simulink library "RCD2"  (R2025b)
settings: Solver=VariableStepAuto  StartTime=0.0  StopTime=10.0  RelTol=1e-3
libraries: simulink x73, etargetslib x4, $bdroot x2
(part 2 of 2)

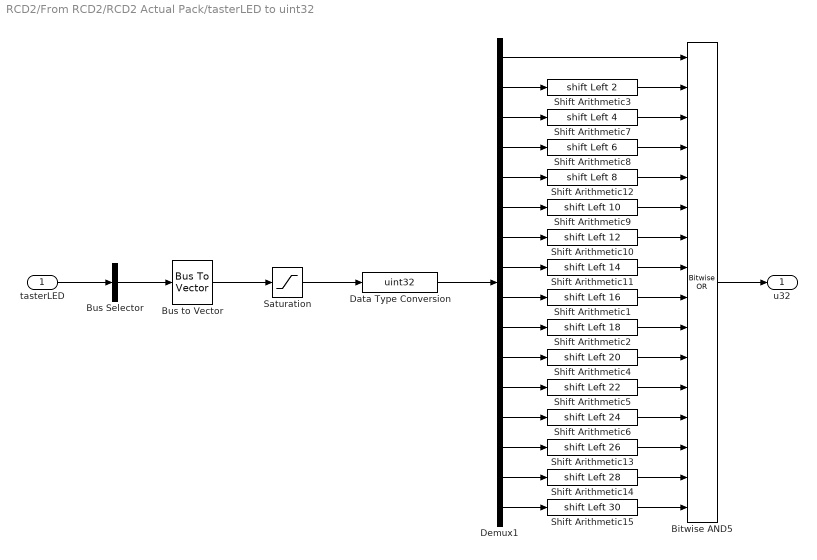
== system RCD2/From RCD2/RCD2 Actual Pack/tasterLED to uint32 ==
  "tasterLED " : Inport
  Bitwise AND5 : simulink/Logic and Bit Operations/Bitwise Operator  logicop=OR  UseBitMask=off  NumInputPorts=16  BitMask=bin2dec('11011001')  BitMaskRealWorld=Stored Integer
      settings: LibrarySourceBlock=|
      | simulink/Quick Insert/Logic and Bit
      | Operations/Bitwise AND
  Bus Selector : BusSelector  OutputSignals=tasterLED1,tasterLED2,tasterLED3,tasterLED4,tasterLED5,tasterLED6,tasterLED7,tasterLED8,tasterLED9,tasterLED10,tasterLED11,tasterLED12,tasterLED13,tasterLED14,tasterLED15,tasterLED16  OutputAsBus=on
  Bus to Vector : BusToVector
  Data Type Conversion : DataTypeConversion  OutDataTypeStr=uint32  SaturateOnIntegerOverflow=off  RndMeth=Floor
  Demux1 : Demux  Outputs=16
  Saturation : Saturate  UpperLimit=uint8(3)  LowerLimit=uint8(0)
  Shift Arithmetic1 : ArithShift  BitShiftNumber=16  BitShiftDirection=Left
  Shift Arithmetic10 : ArithShift  BitShiftNumber=12  BitShiftDirection=Left
  Shift Arithmetic11 : ArithShift  BitShiftNumber=14  BitShiftDirection=Left
  Shift Arithmetic12 : ArithShift  BitShiftNumber=8  BitShiftDirection=Left
  Shift Arithmetic13 : ArithShift  BitShiftNumber=26  BitShiftDirection=Left
  Shift Arithmetic14 : ArithShift  BitShiftNumber=28  BitShiftDirection=Left
  Shift Arithmetic15 : ArithShift  BitShiftNumber=30  BitShiftDirection=Left
  Shift Arithmetic2 : ArithShift  BitShiftNumber=18  BitShiftDirection=Left
  Shift Arithmetic3 : ArithShift  BitShiftNumber=2  BitShiftDirection=Left
  Shift Arithmetic4 : ArithShift  BitShiftNumber=20  BitShiftDirection=Left
  Shift Arithmetic5 : ArithShift  BitShiftNumber=22  BitShiftDirection=Left
  Shift Arithmetic6 : ArithShift  BitShiftNumber=24  BitShiftDirection=Left
  Shift Arithmetic7 : ArithShift  BitShiftNumber=4  BitShiftDirection=Left
  Shift Arithmetic8 : ArithShift  BitShiftNumber=6  BitShiftDirection=Left
  Shift Arithmetic9 : ArithShift  BitShiftNumber=10  BitShiftDirection=Left
  u32 : Outport
  wires:
  Bitwise AND5/1 -> u32/1
  Demux1/6 -> Shift Arithmetic9/1
  Demux1/5 -> Shift Arithmetic12/1
  Shift Arithmetic11/1 -> Bitwise AND5/8
  Shift Arithmetic10/1 -> Bitwise AND5/7
  Demux1/1 -> Bitwise AND5/1
  Shift Arithmetic9/1 -> Bitwise AND5/6
  Shift Arithmetic3/1 -> Bitwise AND5/2
  Demux1/8 -> Shift Arithmetic11/1
  Shift Arithmetic12/1 -> Bitwise AND5/5
  Shift Arithmetic7/1 -> Bitwise AND5/3
  Demux1/7 -> Shift Arithmetic10/1
  Demux1/3 -> Shift Arithmetic7/1
  Demux1/2 -> Shift Arithmetic3/1
  Demux1/4 -> Shift Arithmetic8/1
  Shift Arithmetic8/1 -> Bitwise AND5/4
  Demux1/9 -> Shift Arithmetic1/1
  Shift Arithmetic1/1 -> Bitwise AND5/9
  Demux1/10 -> Shift Arithmetic2/1
  Demux1/11 -> Shift Arithmetic4/1
  Shift Arithmetic2/1 -> Bitwise AND5/10
  Shift Arithmetic4/1 -> Bitwise AND5/11
  Demux1/12 -> Shift Arithmetic5/1
  Shift Arithmetic5/1 -> Bitwise AND5/12
  Demux1/13 -> Shift Arithmetic6/1
  Shift Arithmetic6/1 -> Bitwise AND5/13
  Shift Arithmetic13/1 -> Bitwise AND5/14
  Demux1/14 -> Shift Arithmetic13/1
  Shift Arithmetic14/1 -> Bitwise AND5/15
  Demux1/15 -> Shift Arithmetic14/1
  Shift Arithmetic15/1 -> Bitwise AND5/16
  Demux1/16 -> Shift Arithmetic15/1
  "tasterLED "/1 -> Bus Selector/1
  Bus Selector/1 -> Bus to Vector/1
  Bus to Vector/1 -> Saturation/1
  Data Type Conversion/1 -> Demux1/1
  Saturation/1 -> Data Type Conversion/1

== system RCD2/From RCD2/RCD2 Actual Unpack/Unpack Message ==
  bytes : Inport
  Enable : EnablePort
  Byte Unpack : etargetslib/Byte Unpack  dimensions={4,1,1,1,1,1,1,1,1,1,1,1}  datatypes={'uint8','uint8','double','single','single','single','single','single','single','uint16','uint32','uint16'}  byteAlign=1
      settings: LibrarySourceBlock=embeddedtargetslib/Host Communication/Byte Unpack
  CheckForValidProtocol : Subsystem
  Data Type Conversion{,1..5} (6 alike) : DataTypeConversion  OutDataTypeStr=double  SaturateOnIntegerOverflow=off  RndMeth=Floor
  Selector : Selector  IndexOptions=Index vector (dialog)  Indices=1:45  OutputSizes=1
  Subsystem : Subsystem
  u16 to bitfield : Subsystem
  u16 to tasterBitfield : Subsystem
  u32 to bitfield : Subsystem
  success : Outport
  busRCDActual : Outport  Port=2
  wires:
  bytes/1 -> Selector/1
  CheckForValidProtocol/1(isValid) -> success/1, Subsystem/Enable
  Subsystem/1(Out1) -> busRCDActual/1
  Data Type Conversion/1 -> Subsystem/2(In3)
  Data Type Conversion1/1 -> Subsystem/3(In4)
  Data Type Conversion2/1 -> Subsystem/4(In5)
  Data Type Conversion3/1 -> Subsystem/5(In6)
  Data Type Conversion4/1 -> Subsystem/6(In7)
  Data Type Conversion5/1 -> Subsystem/7(In8)
  u16 to tasterBitfield/1("tasterBitfield ") -> Subsystem/8(In9)
  u32 to bitfield/1("bitfield ") -> Subsystem/9(In10)
  u16 to bitfield/1("bitfield ") -> Subsystem/10(In11)
  Selector/1 -> Byte Unpack/1
  Byte Unpack/2 -> CheckForValidProtocol/2(headerID)
  Byte Unpack/1 -> CheckForValidProtocol/1(headerRCD)
  Byte Unpack/3 -> Subsystem/1(In1)
  Byte Unpack/4 -> Data Type Conversion/1
  Byte Unpack/5 -> Data Type Conversion1/1
  Byte Unpack/6 -> Data Type Conversion2/1
  Byte Unpack/7 -> Data Type Conversion3/1
  Byte Unpack/8 -> Data Type Conversion4/1
  Byte Unpack/9 -> Data Type Conversion5/1
  Byte Unpack/10 -> u16 to tasterBitfield/1(u16)
  Byte Unpack/11 -> u32 to bitfield/1(u32)
  Byte Unpack/12 -> u16 to bitfield/1(u16)

== system RCD2/To RCD2/RCD2 Command Pack/LED to uint16 ==
  "LED " : Inport
  Bitwise AND5 : simulink/Logic and Bit Operations/Bitwise Operator  logicop=OR  UseBitMask=off  NumInputPorts=8  BitMask=bin2dec('11011001')  BitMaskRealWorld=Stored Integer
      settings: LibrarySourceBlock=|
      | simulink/Quick Insert/Logic and Bit
      | Operations/Bitwise AND
  Bus Selector : BusSelector  OutputSignals=LED1,LED2,LED3,LED4,LED5,LED6,LED7,LED8  OutputAsBus=on
  Bus to Vector : BusToVector
  Data Type Conversion : DataTypeConversion  OutDataTypeStr=uint16  SaturateOnIntegerOverflow=off  RndMeth=Floor
  Demux1 : Demux  Outputs=8
  Saturation : Saturate  UpperLimit=uint8(3)  LowerLimit=uint8(0)
  Shift Arithmetic10 : ArithShift  BitShiftNumber=12  BitShiftDirection=Left
  Shift Arithmetic11 : ArithShift  BitShiftNumber=14  BitShiftDirection=Left
  Shift Arithmetic12 : ArithShift  BitShiftNumber=8  BitShiftDirection=Left
  Shift Arithmetic3 : ArithShift  BitShiftNumber=2  BitShiftDirection=Left
  Shift Arithmetic7 : ArithShift  BitShiftNumber=4  BitShiftDirection=Left
  Shift Arithmetic8 : ArithShift  BitShiftNumber=6  BitShiftDirection=Left
  Shift Arithmetic9 : ArithShift  BitShiftNumber=10  BitShiftDirection=Left
  u16 : Outport
  wires:
  Shift Arithmetic8/1 -> Bitwise AND5/4
  Demux1/4 -> Shift Arithmetic8/1
  Demux1/2 -> Shift Arithmetic3/1
  Demux1/3 -> Shift Arithmetic7/1
  Demux1/7 -> Shift Arithmetic10/1
  Shift Arithmetic7/1 -> Bitwise AND5/3
  Shift Arithmetic12/1 -> Bitwise AND5/5
  Demux1/8 -> Shift Arithmetic11/1
  Shift Arithmetic3/1 -> Bitwise AND5/2
  Shift Arithmetic9/1 -> Bitwise AND5/6
  Demux1/1 -> Bitwise AND5/1
  Shift Arithmetic10/1 -> Bitwise AND5/7
  Shift Arithmetic11/1 -> Bitwise AND5/8
  Demux1/5 -> Shift Arithmetic12/1
  Demux1/6 -> Shift Arithmetic9/1
  Bitwise AND5/1 -> u16/1
  "LED "/1 -> Bus Selector/1
  Bus Selector/1 -> Bus to Vector/1
  Bus to Vector/1 -> Saturation/1
  Data Type Conversion/1 -> Demux1/1
  Saturation/1 -> Data Type Conversion/1

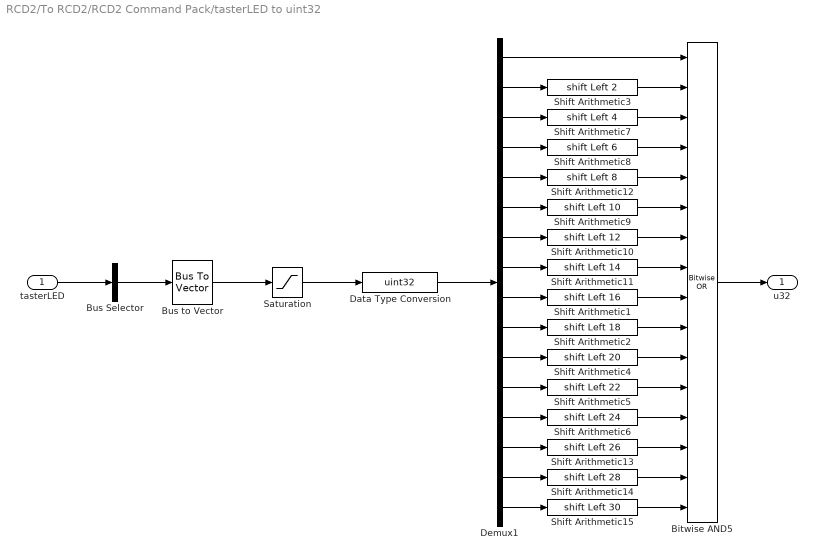
== system RCD2/To RCD2/RCD2 Command Pack/tasterLED to uint32 ==
  "tasterLED " : Inport
  Bitwise AND5 : simulink/Logic and Bit Operations/Bitwise Operator  logicop=OR  UseBitMask=off  NumInputPorts=16  BitMask=bin2dec('11011001')  BitMaskRealWorld=Stored Integer
      settings: LibrarySourceBlock=|
      | simulink/Quick Insert/Logic and Bit
      | Operations/Bitwise AND
  Bus Selector : BusSelector  OutputSignals=tasterLED1,tasterLED2,tasterLED3,tasterLED4,tasterLED5,tasterLED6,tasterLED7,tasterLED8,tasterLED9,tasterLED10,tasterLED11,tasterLED12,tasterLED13,tasterLED14,tasterLED15,tasterLED16  OutputAsBus=on
  Bus to Vector : BusToVector
  Data Type Conversion : DataTypeConversion  OutDataTypeStr=uint32  SaturateOnIntegerOverflow=off  RndMeth=Floor
  Demux1 : Demux  Outputs=16
  Saturation : Saturate  UpperLimit=uint8(3)  LowerLimit=uint8(0)
  Shift Arithmetic1 : ArithShift  BitShiftNumber=16  BitShiftDirection=Left
  Shift Arithmetic10 : ArithShift  BitShiftNumber=12  BitShiftDirection=Left
  Shift Arithmetic11 : ArithShift  BitShiftNumber=14  BitShiftDirection=Left
  Shift Arithmetic12 : ArithShift  BitShiftNumber=8  BitShiftDirection=Left
  Shift Arithmetic13 : ArithShift  BitShiftNumber=26  BitShiftDirection=Left
  Shift Arithmetic14 : ArithShift  BitShiftNumber=28  BitShiftDirection=Left
  Shift Arithmetic15 : ArithShift  BitShiftNumber=30  BitShiftDirection=Left
  Shift Arithmetic2 : ArithShift  BitShiftNumber=18  BitShiftDirection=Left
  Shift Arithmetic3 : ArithShift  BitShiftNumber=2  BitShiftDirection=Left
  Shift Arithmetic4 : ArithShift  BitShiftNumber=20  BitShiftDirection=Left
  Shift Arithmetic5 : ArithShift  BitShiftNumber=22  BitShiftDirection=Left
  Shift Arithmetic6 : ArithShift  BitShiftNumber=24  BitShiftDirection=Left
  Shift Arithmetic7 : ArithShift  BitShiftNumber=4  BitShiftDirection=Left
  Shift Arithmetic8 : ArithShift  BitShiftNumber=6  BitShiftDirection=Left
  Shift Arithmetic9 : ArithShift  BitShiftNumber=10  BitShiftDirection=Left
  u32 : Outport
  wires:
  Bitwise AND5/1 -> u32/1
  Demux1/6 -> Shift Arithmetic9/1
  Demux1/5 -> Shift Arithmetic12/1
  Shift Arithmetic11/1 -> Bitwise AND5/8
  Shift Arithmetic10/1 -> Bitwise AND5/7
  Demux1/1 -> Bitwise AND5/1
  Shift Arithmetic9/1 -> Bitwise AND5/6
  Shift Arithmetic3/1 -> Bitwise AND5/2
  Demux1/8 -> Shift Arithmetic11/1
  Shift Arithmetic12/1 -> Bitwise AND5/5
  Shift Arithmetic7/1 -> Bitwise AND5/3
  Demux1/7 -> Shift Arithmetic10/1
  Demux1/3 -> Shift Arithmetic7/1
  Demux1/2 -> Shift Arithmetic3/1
  Demux1/4 -> Shift Arithmetic8/1
  Shift Arithmetic8/1 -> Bitwise AND5/4
  Demux1/9 -> Shift Arithmetic1/1
  Shift Arithmetic1/1 -> Bitwise AND5/9
  Demux1/10 -> Shift Arithmetic2/1
  Demux1/11 -> Shift Arithmetic4/1
  Shift Arithmetic2/1 -> Bitwise AND5/10
  Shift Arithmetic4/1 -> Bitwise AND5/11
  Demux1/12 -> Shift Arithmetic5/1
  Shift Arithmetic5/1 -> Bitwise AND5/12
  Demux1/13 -> Shift Arithmetic6/1
  Shift Arithmetic6/1 -> Bitwise AND5/13
  Shift Arithmetic13/1 -> Bitwise AND5/14
  Demux1/14 -> Shift Arithmetic13/1
  Shift Arithmetic14/1 -> Bitwise AND5/15
  Demux1/15 -> Shift Arithmetic14/1
  Shift Arithmetic15/1 -> Bitwise AND5/16
  Demux1/16 -> Shift Arithmetic15/1
  "tasterLED "/1 -> Bus Selector/1
  Bus Selector/1 -> Bus to Vector/1
  Bus to Vector/1 -> Saturation/1
  Data Type Conversion/1 -> Demux1/1
  Saturation/1 -> Data Type Conversion/1

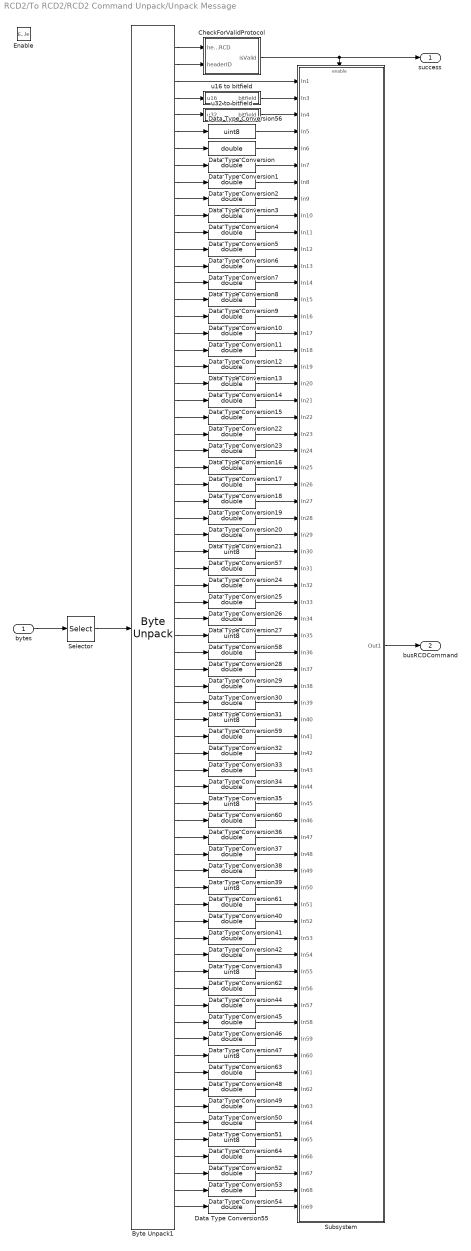
== system RCD2/To RCD2/RCD2 Command Unpack/Unpack Message ==
  bytes : Inport
  Enable : EnablePort
  Byte Unpack1 : etargetslib/Byte Unpack  dimensions={4,1,1,1,1,16,1,1,1,1,1,1,1,1,1,1,1,1,1,1,1,1,1,1,1,1,1,1,1,1,8,1,1,1,1,8,1,1,1,1,8,1,1,1,1,8,1,1,1,1,8,1,1,1,1,8,1,1,1,1,8,1,1,1,1,8,1,1,1,1}  datatypes={'uint8', 'uint8','double','uint16','uint32','uint8','single','single','single','single','single','single','single','single','single','single','single','single','single','single','single','single','single','single','single','single','single','single','single','single','uint8','single','single','single','single','uint8','single','single','single','single','uint8','single','single','single','single','uint8','single','single','single','single','uint8','single','single','single','single','uint8','single','single','single','single','uint8','single','single','single','single','uint8','single','single','single','single'}  byteAlign=1
      settings: LibrarySourceBlock=embeddedtargetslib/Host Communication/Byte Unpack
  CheckForValidProtocol : Subsystem
  Data Type Conversion{,1..55} (56 alike) : DataTypeConversion  OutDataTypeStr=double  SaturateOnIntegerOverflow=off  RndMeth=Floor
  Data Type Conversion{56..64} (9 alike) : DataTypeConversion  OutDataTypeStr=uint8  SaturateOnIntegerOverflow=off  RndMeth=Floor
  Selector : Selector  IndexOptions=Index vector (dialog)  Indices=1:323  OutputSizes=1
  Subsystem : Subsystem
  u16 to bitfield : Subsystem
  u32 to bitfield : Subsystem
  success : Outport
  busRCDCommand : Outport  Port=2
  wires:
  Byte Unpack1/66 -> Data Type Conversion64/1
  Byte Unpack1/5 -> u32 to bitfield/1(u32)
  Byte Unpack1/56 -> Data Type Conversion62/1
  Byte Unpack1/36 -> Data Type Conversion58/1
  Byte Unpack1/41 -> Data Type Conversion59/1
  Byte Unpack1/6 -> Data Type Conversion56/1
  Byte Unpack1/61 -> Data Type Conversion63/1
  Byte Unpack1/51 -> Data Type Conversion61/1
  Byte Unpack1/46 -> Data Type Conversion60/1
  Byte Unpack1/2 -> CheckForValidProtocol/2(headerID)
  Byte Unpack1/31 -> Data Type Conversion57/1
  bytes/1 -> Selector/1
  Byte Unpack1/7 -> Data Type Conversion/1
  Byte Unpack1/8 -> Data Type Conversion1/1
  Byte Unpack1/10 -> Data Type Conversion3/1
  Byte Unpack1/9 -> Data Type Conversion2/1
  Byte Unpack1/13 -> Data Type Conversion6/1
  Byte Unpack1/14 -> Data Type Conversion7/1
  Byte Unpack1/12 -> Data Type Conversion5/1
  Byte Unpack1/11 -> Data Type Conversion4/1
  Byte Unpack1/19 -> Data Type Conversion12/1
  Byte Unpack1/20 -> Data Type Conversion13/1
  Byte Unpack1/22 -> Data Type Conversion15/1
  Byte Unpack1/21 -> Data Type Conversion14/1
  Byte Unpack1/17 -> Data Type Conversion10/1
  Byte Unpack1/18 -> Data Type Conversion11/1
  Byte Unpack1/16 -> Data Type Conversion9/1
  Byte Unpack1/15 -> Data Type Conversion8/1
  Byte Unpack1/23 -> Data Type Conversion22/1
  Byte Unpack1/24 -> Data Type Conversion23/1
  Byte Unpack1/26 -> Data Type Conversion17/1
  Byte Unpack1/25 -> Data Type Conversion16/1
  Byte Unpack1/29 -> Data Type Conversion20/1
  Byte Unpack1/30 -> Data Type Conversion21/1
  Byte Unpack1/28 -> Data Type Conversion19/1
  Byte Unpack1/27 -> Data Type Conversion18/1
  Byte Unpack1/32 -> Data Type Conversion24/1
  Byte Unpack1/33 -> Data Type Conversion25/1
  Byte Unpack1/35 -> Data Type Conversion27/1
  Byte Unpack1/34 -> Data Type Conversion26/1
  Byte Unpack1/39 -> Data Type Conversion30/1
  Byte Unpack1/40 -> Data Type Conversion31/1
  Byte Unpack1/38 -> Data Type Conversion29/1
  Byte Unpack1/37 -> Data Type Conversion28/1
  Byte Unpack1/42 -> Data Type Conversion32/1
  Byte Unpack1/43 -> Data Type Conversion33/1
  Byte Unpack1/45 -> Data Type Conversion35/1
  Byte Unpack1/44 -> Data Type Conversion34/1
  Byte Unpack1/49 -> Data Type Conversion38/1
  Byte Unpack1/50 -> Data Type Conversion39/1
  Byte Unpack1/48 -> Data Type Conversion37/1
  Byte Unpack1/47 -> Data Type Conversion36/1
  Byte Unpack1/52 -> Data Type Conversion40/1
  Byte Unpack1/53 -> Data Type Conversion41/1
  Byte Unpack1/55 -> Data Type Conversion43/1
  Byte Unpack1/54 -> Data Type Conversion42/1
  Byte Unpack1/59 -> Data Type Conversion46/1
  Byte Unpack1/60 -> Data Type Conversion47/1
  Byte Unpack1/58 -> Data Type Conversion45/1
  Byte Unpack1/57 -> Data Type Conversion44/1
  Byte Unpack1/62 -> Data Type Conversion48/1
  Byte Unpack1/63 -> Data Type Conversion49/1
  Byte Unpack1/65 -> Data Type Conversion51/1
  Byte Unpack1/64 -> Data Type Conversion50/1
  Byte Unpack1/69 -> Data Type Conversion54/1
  Byte Unpack1/70 -> Data Type Conversion55/1
  Byte Unpack1/68 -> Data Type Conversion53/1
  Byte Unpack1/67 -> Data Type Conversion52/1
  Byte Unpack1/1 -> CheckForValidProtocol/1(headerRCD)
  CheckForValidProtocol/1(isValid) -> success/1, Subsystem/Enable
  Byte Unpack1/4 -> u16 to bitfield/1(u16)
  u16 to bitfield/1("bitfield ") -> Subsystem/2(In3)
  u32 to bitfield/1("bitfield ") -> Subsystem/3(In4)
  Data Type Conversion56/1 -> Subsystem/4(In5)
  Data Type Conversion/1 -> Subsystem/5(In6)
  Data Type Conversion1/1 -> Subsystem/6(In7)
  Data Type Conversion2/1 -> Subsystem/7(In8)
  Data Type Conversion3/1 -> Subsystem/8(In9)
  Data Type Conversion4/1 -> Subsystem/9(In10)
  Data Type Conversion5/1 -> Subsystem/10(In11)
  Data Type Conversion6/1 -> Subsystem/11(In12)
  Data Type Conversion7/1 -> Subsystem/12(In13)
  Data Type Conversion8/1 -> Subsystem/13(In14)
  Data Type Conversion9/1 -> Subsystem/14(In15)
  Data Type Conversion10/1 -> Subsystem/15(In16)
  Data Type Conversion11/1 -> Subsystem/16(In17)
  Data Type Conversion12/1 -> Subsystem/17(In18)
  Data Type Conversion13/1 -> Subsystem/18(In19)
  Data Type Conversion14/1 -> Subsystem/19(In20)
  Data Type Conversion15/1 -> Subsystem/20(In21)
  Data Type Conversion22/1 -> Subsystem/21(In22)
  Data Type Conversion23/1 -> Subsystem/22(In23)
  Data Type Conversion16/1 -> Subsystem/23(In24)
  Data Type Conversion17/1 -> Subsystem/24(In25)
  Data Type Conversion18/1 -> Subsystem/25(In26)
  Data Type Conversion19/1 -> Subsystem/26(In27)
  Data Type Conversion20/1 -> Subsystem/27(In28)
  Data Type Conversion21/1 -> Subsystem/28(In29)
  Data Type Conversion57/1 -> Subsystem/29(In30)
  Data Type Conversion24/1 -> Subsystem/30(In31)
  Data Type Conversion25/1 -> Subsystem/31(In32)
  Data Type Conversion26/1 -> Subsystem/32(In33)
  Data Type Conversion27/1 -> Subsystem/33(In34)
  Data Type Conversion58/1 -> Subsystem/34(In35)
  Data Type Conversion28/1 -> Subsystem/35(In36)
  Data Type Conversion29/1 -> Subsystem/36(In37)
  Data Type Conversion30/1 -> Subsystem/37(In38)
  Data Type Conversion31/1 -> Subsystem/38(In39)
  Data Type Conversion59/1 -> Subsystem/39(In40)
  Data Type Conversion32/1 -> Subsystem/40(In41)
  Data Type Conversion33/1 -> Subsystem/41(In42)
  Data Type Conversion34/1 -> Subsystem/42(In43)
  Data Type Conversion35/1 -> Subsystem/43(In44)
  Data Type Conversion60/1 -> Subsystem/44(In45)
  Data Type Conversion36/1 -> Subsystem/45(In46)
  Data Type Conversion37/1 -> Subsystem/46(In47)
  Data Type Conversion38/1 -> Subsystem/47(In48)
  Data Type Conversion39/1 -> Subsystem/48(In49)
  Data Type Conversion61/1 -> Subsystem/49(In50)
  Data Type Conversion40/1 -> Subsystem/50(In51)
  Data Type Conversion41/1 -> Subsystem/51(In52)
  Data Type Conversion42/1 -> Subsystem/52(In53)
  Data Type Conversion43/1 -> Subsystem/53(In54)
  Data Type Conversion62/1 -> Subsystem/54(In55)
  Data Type Conversion44/1 -> Subsystem/55(In56)
  Data Type Conversion45/1 -> Subsystem/56(In57)
  Data Type Conversion46/1 -> Subsystem/57(In58)
  Data Type Conversion47/1 -> Subsystem/58(In59)
  Data Type Conversion63/1 -> Subsystem/59(In60)
  Data Type Conversion48/1 -> Subsystem/60(In61)
  Data Type Conversion49/1 -> Subsystem/61(In62)
  Data Type Conversion50/1 -> Subsystem/62(In63)
  Data Type Conversion51/1 -> Subsystem/63(In64)
  Data Type Conversion64/1 -> Subsystem/64(In65)
  Data Type Conversion52/1 -> Subsystem/65(In66)
  Data Type Conversion53/1 -> Subsystem/66(In67)
  Data Type Conversion54/1 -> Subsystem/67(In68)
  Data Type Conversion55/1 -> Subsystem/68(In69)
  Subsystem/1(Out1) -> busRCDCommand/1
  Byte Unpack1/3 -> Subsystem/1(In1)
  Selector/1 -> Byte Unpack1/1

== system RCD2/From RCD2/RCD2 Actual Unpack/Unpack Message/CheckForValidProtocol ==
  headerRCD : Inport
  headerID : Inport  Port=2
  AND : Logic  AllPortsSameDT=off  OutDataTypeStr=boolean
  ASCII to String10 : ASCIIToString
  Compare To Constant : simulink/Logic and Bit Operations/Compare To Constant  relop===  const=uint8(idRCD)  OutDataTypeStr=boolean
  String Compare : StringCompare
  String Constant : StringConstant  String="\"RCD2\""
  isValid : Outport  OutDataTypeStr=boolean  PortDimensions=1
  wires:
  String Constant/1 -> String Compare/1
  headerRCD/1 -> ASCII to String10/1
  headerID/1 -> Compare To Constant/1
  Compare To Constant/1 -> AND/2
  String Compare/1 -> AND/1
  AND/1 -> isValid/1
  ASCII to String10/1 -> String Compare/2

== system RCD2/From RCD2/RCD2 Actual Unpack/Unpack Message/Subsystem ==
  In1 : Inport
  In3 : Inport  Port=2
  In4 : Inport  Port=3
  In5 : Inport  Port=4
  In6 : Inport  Port=5
  In7 : Inport  Port=6
  In8 : Inport  Port=7
  In9 : Inport  Port=8
  In10 : Inport  Port=9
  In11 : Inport  Port=10
  Enable : EnablePort
  Bus Assignment : BusAssignment  AssignedSignals=timestamp,joystick.joystickX,joystick.joystickY,joystick.joystickZ,potentiometer.potentiometer1,potentiometer.potentiometer2,potentiometer.potentiometer3,taster.taster1,taster.taster2,taster.taster3,taster.taster4,taster.taster5,taster.taster6,taster.taster7,taster.taster8,taster.taster9,taster.taster10,taster.taster11,taster.taster12,taster.taster13,taster.taster14,taster.taster15,taster.taster16,tasterLED.tasterLED1,tasterLED.tasterLED2,tasterLED.tasterLED3,tasterLED.tasterLED4,tasterLED.tasterLED5,tasterLED.tasterLED6,tasterLED.tasterLED7,tasterLED.tasterLED8,tasterLED.tasterLED9,tasterLED.tasterLED10,tasterLED.tasterLED11,tasterLED.tasterLED12,tasterLED.tasterLED13,tasterLED.tasterLED14,tasterLED.tasterLED15,tasterLED.tasterLED16,LED.LED1,LED.LED2,LED.LED3,LED.LED4,LED.LED5,LED.LED6,LED.LED7,LED.LED8
  Demux : Demux  Outputs=8
  Demux1 : Demux  Outputs=16
  Demux2 : Demux  Outputs=16
  RCD2 Actual Empty Bus : $bdroot/From RCD2/RCD2 Actual Empty Bus
  Out1 : Outport
  wires:
  Demux2/6 -> Bus Assignment/30
  Demux1/4 -> Bus Assignment/12
  Demux1/14 -> Bus Assignment/22
  Demux1/7 -> Bus Assignment/15
  Demux2/16 -> Bus Assignment/40
  In4/1 -> Bus Assignment/4
  Demux2/14 -> Bus Assignment/38
  Demux/8 -> Bus Assignment/48
  Demux1/6 -> Bus Assignment/14
  Demux2/15 -> Bus Assignment/39
  Demux2/8 -> Bus Assignment/32
  Demux/1 -> Bus Assignment/41
  Demux2/9 -> Bus Assignment/33
  Demux2/10 -> Bus Assignment/34
  Demux2/13 -> Bus Assignment/37
  Demux1/2 -> Bus Assignment/10
  Demux1/15 -> Bus Assignment/23
  Demux1/12 -> Bus Assignment/20
  Demux2/11 -> Bus Assignment/35
  Demux/5 -> Bus Assignment/45
  Demux2/7 -> Bus Assignment/31
  In3/1 -> Bus Assignment/3
  In8/1 -> Bus Assignment/8
  Demux1/13 -> Bus Assignment/21
  Bus Assignment/1 -> Out1/1
  Demux/6 -> Bus Assignment/46
  In1/1 -> Bus Assignment/2
  Demux1/16 -> Bus Assignment/24
  In7/1 -> Bus Assignment/7
  Demux1/5 -> Bus Assignment/13
  In6/1 -> Bus Assignment/6
  Demux1/11 -> Bus Assignment/19
  Demux/2 -> Bus Assignment/42
  In11/1 -> Demux/1
  Demux1/1 -> Bus Assignment/9
  Demux1/3 -> Bus Assignment/11
  Demux2/2 -> Bus Assignment/26
  In5/1 -> Bus Assignment/5
  Demux1/10 -> Bus Assignment/18
  RCD2 Actual Empty Bus/1 -> Bus Assignment/1
  Demux/3 -> Bus Assignment/43
  Demux/7 -> Bus Assignment/47
  In9/1 -> Demux1/1
  Demux2/3 -> Bus Assignment/27
  In10/1 -> Demux2/1
  Demux1/8 -> Bus Assignment/16
  Demux2/1 -> Bus Assignment/25
  Demux2/4 -> Bus Assignment/28
  Demux2/5 -> Bus Assignment/29
  Demux2/12 -> Bus Assignment/36
  Demux/4 -> Bus Assignment/44
  Demux1/9 -> Bus Assignment/17

== system RCD2/From RCD2/RCD2 Actual Unpack/Unpack Message/u16 to bitfield ==
  u16 : Inport
  Bitwise AND{6,10..16} (8 alike) : simulink/Logic and Bit Operations/Bitwise Operator  logicop=AND  UseBitMask=on  BitMask=3  BitMaskRealWorld=Stored Integer
      settings: LibrarySourceBlock=|
      | simulink/Quick Insert/Logic and Bit
      | Operations/Bitwise AND
  Data Type Conversion5 : DataTypeConversion  OutDataTypeStr=uint8  SaturateOnIntegerOverflow=off  RndMeth=Floor
  Mux : Mux  Inputs=8
  Shift Arithmetic16 : ArithShift  BitShiftNumber=2  BitShiftDirection=Right
  Shift Arithmetic17 : ArithShift  BitShiftNumber=4  BitShiftDirection=Right
  Shift Arithmetic18 : ArithShift  BitShiftNumber=6  BitShiftDirection=Right
  Shift Arithmetic19 : ArithShift  BitShiftNumber=8  BitShiftDirection=Right
  Shift Arithmetic20 : ArithShift  BitShiftNumber=10  BitShiftDirection=Right
  Shift Arithmetic21 : ArithShift  BitShiftNumber=12  BitShiftDirection=Right
  Shift Arithmetic22 : ArithShift  BitShiftNumber=14  BitShiftDirection=Right
  "bitfield " : Outport
  wires:
  Mux/1 -> Data Type Conversion5/1
  Shift Arithmetic20/1 -> Bitwise AND14/1
  Shift Arithmetic19/1 -> Bitwise AND13/1
  Shift Arithmetic17/1 -> Bitwise AND11/1
  Shift Arithmetic16/1 -> Bitwise AND10/1
  Shift Arithmetic21/1 -> Bitwise AND15/1
  Shift Arithmetic22/1 -> Bitwise AND16/1
  Shift Arithmetic18/1 -> Bitwise AND12/1
  u16/1 -> Shift Arithmetic16/1, Shift Arithmetic17/1, Shift Arithmetic18/1, Shift Arithmetic19/1, Shift Arithmetic20/1, Shift Arithmetic21/1, Shift Arithmetic22/1, Bitwise AND6/1
  Bitwise AND6/1 -> Mux/1
  Bitwise AND10/1 -> Mux/2
  Bitwise AND11/1 -> Mux/3
  Bitwise AND12/1 -> Mux/4
  Bitwise AND13/1 -> Mux/5
  Bitwise AND14/1 -> Mux/6
  Bitwise AND15/1 -> Mux/7
  Bitwise AND16/1 -> Mux/8
  Data Type Conversion5/1 -> "bitfield "/1

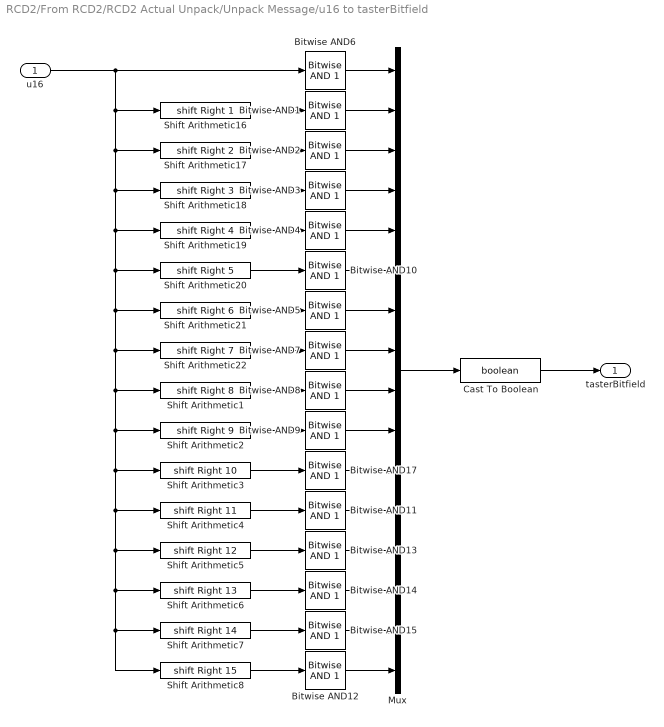
== system RCD2/From RCD2/RCD2 Actual Unpack/Unpack Message/u16 to tasterBitfield ==
  u16 : Inport
  Bitwise AND{1..15,17} (16 alike) : simulink/Logic and Bit Operations/Bitwise Operator  logicop=AND  UseBitMask=on  BitMask=1  BitMaskRealWorld=Stored Integer
      settings: LibrarySourceBlock=|
      | simulink/Quick Insert/Logic and Bit
      | Operations/Bitwise AND
  Cast To Boolean : DataTypeConversion  OutDataTypeStr=boolean  SaturateOnIntegerOverflow=off  RndMeth=Floor
  Mux : Mux  Inputs=16
  Shift Arithmetic1 : ArithShift  BitShiftNumber=8  BitShiftDirection=Right
  Shift Arithmetic16 : ArithShift  BitShiftNumber=1  BitShiftDirection=Right
  Shift Arithmetic17 : ArithShift  BitShiftNumber=2  BitShiftDirection=Right
  Shift Arithmetic18 : ArithShift  BitShiftNumber=3  BitShiftDirection=Right
  Shift Arithmetic19 : ArithShift  BitShiftNumber=4  BitShiftDirection=Right
  Shift Arithmetic2 : ArithShift  BitShiftNumber=9  BitShiftDirection=Right
  Shift Arithmetic20 : ArithShift  BitShiftNumber=5  BitShiftDirection=Right
  Shift Arithmetic21 : ArithShift  BitShiftNumber=6  BitShiftDirection=Right
  Shift Arithmetic22 : ArithShift  BitShiftNumber=7  BitShiftDirection=Right
  Shift Arithmetic3 : ArithShift  BitShiftNumber=10  BitShiftDirection=Right
  Shift Arithmetic4 : ArithShift  BitShiftNumber=11  BitShiftDirection=Right
  Shift Arithmetic5 : ArithShift  BitShiftNumber=12  BitShiftDirection=Right
  Shift Arithmetic6 : ArithShift  BitShiftNumber=13  BitShiftDirection=Right
  Shift Arithmetic7 : ArithShift  BitShiftNumber=14  BitShiftDirection=Right
  Shift Arithmetic8 : ArithShift  BitShiftNumber=15  BitShiftDirection=Right
  "tasterBitfield " : Outport
  wires:
  Cast To Boolean/1 -> "tasterBitfield "/1
  Bitwise AND15/1 -> Mux/15
  Bitwise AND14/1 -> Mux/14
  Bitwise AND13/1 -> Mux/13
  Bitwise AND11/1 -> Mux/12
  Bitwise AND17/1 -> Mux/11
  Bitwise AND9/1 -> Mux/10
  Bitwise AND8/1 -> Mux/9
  Bitwise AND7/1 -> Mux/8
  Bitwise AND5/1 -> Mux/7
  Bitwise AND10/1 -> Mux/6
  Bitwise AND4/1 -> Mux/5
  Bitwise AND3/1 -> Mux/4
  Bitwise AND2/1 -> Mux/3
  Bitwise AND1/1 -> Mux/2
  Bitwise AND6/1 -> Mux/1
  u16/1 -> Bitwise AND6/1, Shift Arithmetic8/1, Shift Arithmetic7/1, Shift Arithmetic6/1, Shift Arithmetic5/1, Shift Arithmetic4/1, Shift Arithmetic3/1, Shift Arithmetic2/1, Shift Arithmetic1/1, Shift Arithmetic22/1, Shift Arithmetic21/1, Shift Arithmetic20/1, Shift Arithmetic19/1, Shift Arithmetic18/1, Shift Arithmetic17/1, Shift Arithmetic16/1
  Shift Arithmetic20/1 -> Bitwise AND10/1
  Shift Arithmetic19/1 -> Bitwise AND4/1
  Shift Arithmetic17/1 -> Bitwise AND2/1
  Shift Arithmetic16/1 -> Bitwise AND1/1
  Shift Arithmetic21/1 -> Bitwise AND5/1
  Shift Arithmetic22/1 -> Bitwise AND7/1
  Shift Arithmetic18/1 -> Bitwise AND3/1
  Shift Arithmetic1/1 -> Bitwise AND8/1
  Shift Arithmetic2/1 -> Bitwise AND9/1
  Shift Arithmetic3/1 -> Bitwise AND17/1
  Shift Arithmetic4/1 -> Bitwise AND11/1
  Shift Arithmetic5/1 -> Bitwise AND13/1
  Shift Arithmetic6/1 -> Bitwise AND14/1
  Shift Arithmetic7/1 -> Bitwise AND15/1
  Shift Arithmetic8/1 -> Bitwise AND12/1
  Bitwise AND12/1 -> Mux/16
  Mux/1 -> Cast To Boolean/1

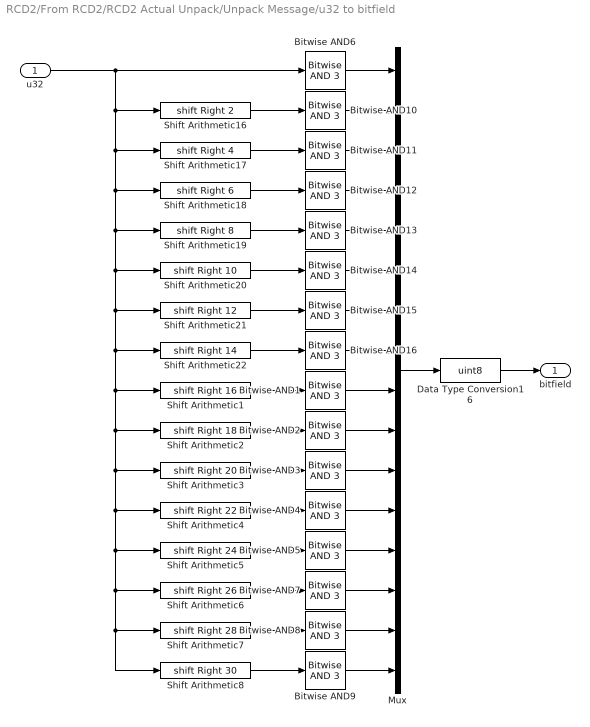
== system RCD2/From RCD2/RCD2 Actual Unpack/Unpack Message/u32 to bitfield ==
  u32 : Inport
  Bitwise AND{1..16} (16 alike) : simulink/Logic and Bit Operations/Bitwise Operator  logicop=AND  UseBitMask=on  BitMask=3  BitMaskRealWorld=Stored Integer
      settings: LibrarySourceBlock=|
      | simulink/Quick Insert/Logic and Bit
      | Operations/Bitwise AND
  Data Type Conversion16 : DataTypeConversion  OutDataTypeStr=uint8  SaturateOnIntegerOverflow=off  RndMeth=Floor
  Mux : Mux  Inputs=16
  Shift Arithmetic1 : ArithShift  BitShiftNumber=16  BitShiftDirection=Right
  Shift Arithmetic16 : ArithShift  BitShiftNumber=2  BitShiftDirection=Right
  Shift Arithmetic17 : ArithShift  BitShiftNumber=4  BitShiftDirection=Right
  Shift Arithmetic18 : ArithShift  BitShiftNumber=6  BitShiftDirection=Right
  Shift Arithmetic19 : ArithShift  BitShiftNumber=8  BitShiftDirection=Right
  Shift Arithmetic2 : ArithShift  BitShiftNumber=18  BitShiftDirection=Right
  Shift Arithmetic20 : ArithShift  BitShiftNumber=10  BitShiftDirection=Right
  Shift Arithmetic21 : ArithShift  BitShiftNumber=12  BitShiftDirection=Right
  Shift Arithmetic22 : ArithShift  BitShiftNumber=14  BitShiftDirection=Right
  Shift Arithmetic3 : ArithShift  BitShiftNumber=20  BitShiftDirection=Right
  Shift Arithmetic4 : ArithShift  BitShiftNumber=22  BitShiftDirection=Right
  Shift Arithmetic5 : ArithShift  BitShiftNumber=24  BitShiftDirection=Right
  Shift Arithmetic6 : ArithShift  BitShiftNumber=26  BitShiftDirection=Right
  Shift Arithmetic7 : ArithShift  BitShiftNumber=28  BitShiftDirection=Right
  Shift Arithmetic8 : ArithShift  BitShiftNumber=30  BitShiftDirection=Right
  "bitfield " : Outport
  wires:
  Mux/1 -> Data Type Conversion16/1
  Bitwise AND9/1 -> Mux/16
  Shift Arithmetic8/1 -> Bitwise AND9/1
  Shift Arithmetic7/1 -> Bitwise AND8/1
  Shift Arithmetic6/1 -> Bitwise AND7/1
  Shift Arithmetic5/1 -> Bitwise AND5/1
  Shift Arithmetic4/1 -> Bitwise AND4/1
  Shift Arithmetic3/1 -> Bitwise AND3/1
  Shift Arithmetic2/1 -> Bitwise AND2/1
  Shift Arithmetic1/1 -> Bitwise AND1/1
  Shift Arithmetic18/1 -> Bitwise AND12/1
  Shift Arithmetic22/1 -> Bitwise AND16/1
  Shift Arithmetic21/1 -> Bitwise AND15/1
  Shift Arithmetic16/1 -> Bitwise AND10/1
  Shift Arithmetic17/1 -> Bitwise AND11/1
  Shift Arithmetic19/1 -> Bitwise AND13/1
  Shift Arithmetic20/1 -> Bitwise AND14/1
  u32/1 -> Shift Arithmetic16/1, Shift Arithmetic17/1, Shift Arithmetic18/1, Shift Arithmetic19/1, Shift Arithmetic20/1, Shift Arithmetic21/1, Shift Arithmetic22/1, Shift Arithmetic1/1, Shift Arithmetic2/1, Shift Arithmetic3/1, Shift Arithmetic4/1, Shift Arithmetic5/1, Shift Arithmetic6/1, Shift Arithmetic7/1, Shift Arithmetic8/1, Bitwise AND6/1
  Bitwise AND6/1 -> Mux/1
  Bitwise AND10/1 -> Mux/2
  Bitwise AND11/1 -> Mux/3
  Bitwise AND12/1 -> Mux/4
  Bitwise AND13/1 -> Mux/5
  Bitwise AND14/1 -> Mux/6
  Bitwise AND15/1 -> Mux/7
  Bitwise AND16/1 -> Mux/8
  Bitwise AND1/1 -> Mux/9
  Bitwise AND2/1 -> Mux/10
  Bitwise AND3/1 -> Mux/11
  Bitwise AND4/1 -> Mux/12
  Bitwise AND5/1 -> Mux/13
  Bitwise AND7/1 -> Mux/14
  Bitwise AND8/1 -> Mux/15
  Data Type Conversion16/1 -> "bitfield "/1

== system RCD2/To RCD2/RCD2 Command Unpack/Unpack Message/CheckForValidProtocol ==
  headerRCD : Inport
  headerID : Inport  Port=2
  AND : Logic  AllPortsSameDT=off  OutDataTypeStr=boolean
  ASCII to String10 : ASCIIToString
  Compare To Constant : simulink/Logic and Bit Operations/Compare To Constant  relop===  const=uint8(idRCD)  OutDataTypeStr=boolean
  String Compare : StringCompare
  String Constant : StringConstant  String="\"RCD2\""
  isValid : Outport  OutDataTypeStr=boolean  PortDimensions=1
  wires:
  String Constant/1 -> String Compare/1
  headerRCD/1 -> ASCII to String10/1
  headerID/1 -> Compare To Constant/1
  Compare To Constant/1 -> AND/2
  String Compare/1 -> AND/1
  AND/1 -> isValid/1
  ASCII to String10/1 -> String Compare/2

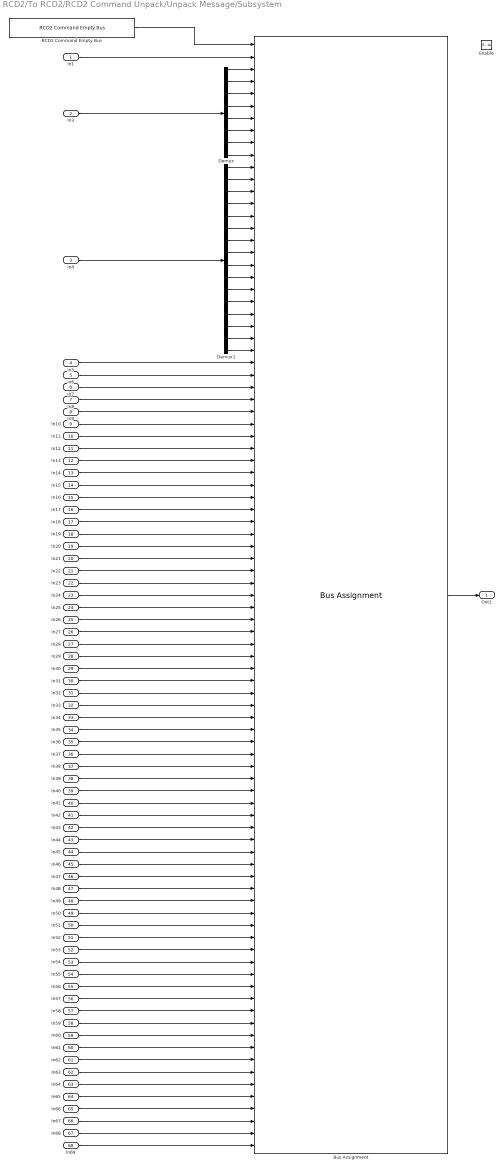
== system RCD2/To RCD2/RCD2 Command Unpack/Unpack Message/Subsystem ==
  In1 : Inport
  In3 : Inport  Port=2
  In4 : Inport  Port=3
  In5 : Inport  Port=4
  In6 : Inport  Port=5
  In7 : Inport  Port=6
  In8 : Inport  Port=7
  In9 : Inport  Port=8
  In10 : Inport  Port=9
  In11 : Inport  Port=10
  In12 : Inport  Port=11
  In13 : Inport  Port=12
  In14 : Inport  Port=13
  In15 : Inport  Port=14
  In16 : Inport  Port=15
  In17 : Inport  Port=16
  In18 : Inport  Port=17
  In19 : Inport  Port=18
  In20 : Inport  Port=19
  In21 : Inport  Port=20
  In22 : Inport  Port=21
  In23 : Inport  Port=22
  In24 : Inport  Port=23
  In25 : Inport  Port=24
  In26 : Inport  Port=25
  In27 : Inport  Port=26
  In28 : Inport  Port=27
  In29 : Inport  Port=28
  In30 : Inport  Port=29
  In31 : Inport  Port=30
  In32 : Inport  Port=31
  In33 : Inport  Port=32
  In34 : Inport  Port=33
  In35 : Inport  Port=34
  In36 : Inport  Port=35
  In37 : Inport  Port=36
  In38 : Inport  Port=37
  In39 : Inport  Port=38
  In40 : Inport  Port=39
  In41 : Inport  Port=40
  In42 : Inport  Port=41
  In43 : Inport  Port=42
  In44 : Inport  Port=43
  In45 : Inport  Port=44
  In46 : Inport  Port=45
  In47 : Inport  Port=46
  In48 : Inport  Port=47
  In49 : Inport  Port=48
  In50 : Inport  Port=49
  In51 : Inport  Port=50
  In52 : Inport  Port=51
  In53 : Inport  Port=52
  In54 : Inport  Port=53
  In55 : Inport  Port=54
  In56 : Inport  Port=55
  In57 : Inport  Port=56
  In58 : Inport  Port=57
  In59 : Inport  Port=58
  In60 : Inport  Port=59
  In61 : Inport  Port=60
  In62 : Inport  Port=61
  In63 : Inport  Port=62
  In64 : Inport  Port=63
  In65 : Inport  Port=64
  In66 : Inport  Port=65
  In67 : Inport  Port=66
  In68 : Inport  Port=67
  In69 : Inport  Port=68
  Enable : EnablePort
  Bus Assignment : BusAssignment  AssignedSignals=timestamp,LED.LED1,LED.LED2,LED.LED3,LED.LED4,LED.LED5,LED.LED6,LED.LED7,LED.LED8,tasterLED.tasterLED1,tasterLED.tasterLED2,tasterLED.tasterLED3,tasterLED.tasterLED4,tasterLED.tasterLED5,tasterLED.tasterLED6,tasterLED.tasterLED7,tasterLED.tasterLED8,tasterLED.tasterLED9,tasterLED.tasterLED10,tasterLED.tasterLED11,tasterLED.tasterLED12,tasterLED.tasterLED13,tasterLED.tasterLED14,tasterLED.tasterLED15,tasterLED.tasterLED16,asciiOperationMode,thrustPlot.displayValues.commandX,thrustPlot.displayValues.commandY,thrustPlot.displayValues.commandN,thrustPlot.displayValues.actualX,thrustPlot.displayValues.actualY,thrustPlot.displayValues.actualN,velocityPlot.displayValues.commandU,velocityPlot.displayValues.commandV,velocityPlot.displayValues.commandR,velocityPlot.displayValues.actualU,velocityPlot.displayValues.actualV,velocityPlot.displayValues.actualR,thrustPlot.normalizedVectorScope.commandAbsoluteValue,thrustPlot.normalizedVectorScope.commandAngle,thrustPlot.normalizedVectorScope.commandZ,thrustPlot.normalizedVectorScope.actualAbsoluteValue,thrustPlot.normalizedVectorScope.actualAngle,thrustPlot.normalizedVectorScope.actualZ,velocityPlot.normalizedVectorScope.commandAbsoluteValue,velocityPlot.normalizedVectorScope.commandAngle,velocityPlot.normalizedVectorScope.commandZ,velocityPlot.normalizedVectorScope.actualAbsoluteValue,velocityPlot.normalizedVectorScope.actualAngle,velocityPlot.normalizedVectorScope.actualZ,actuatorPlot.actuator1.asciiLabel,actuatorPlot.actuator1.normalizedScopeValues.actual,actuatorPlot.actuator1.normalizedScopeValues.command,actuatorPlot.actuator1.displayValues.actual,actuatorPlot.actuator1.displayValues.command,actuatorPlot.actuator2.asciiLabel,actuatorPlot.actuator2.normalizedScopeValues.actual,actuatorPlot.actuator2.normalizedScopeValues.command,actuatorPlot.actuator2.displayValues.actual,actuatorPlot.actuator2.displayValues.command,actuatorPlot.actuator3.asciiLabel,actuatorPlot.actuator3.normalizedScopeValues.actual,actuatorPlot.actuator3.normalizedScopeValues.command,actuatorPlot.actuator3.displayValues.actual,actuatorPlot.actuator3.displayValues.command,actuatorPlot.actuator4.asciiLabel,actuatorPlot.actuator4.normalizedScopeValues.actual,actuatorPlot.actuator4.normalizedScopeValues.command,actuatorPlot.actuator4.displayValues.actual,actuatorPlot.actuator4.displayValues.command,actuatorPlot.actuator5.asciiLabel,actuatorPlot.actuator5.normalizedScopeValues.actual,actuatorPlot.actuator5.normalizedScopeValues.command,actuatorPlot.actuator5.displayValues.actual,actuatorPlot.actuator5.displayValues.command,actuatorPlot.actuator6.asciiLabel,actuatorPlot.actuator6.normalizedScopeValues.actual,actuatorPlot.actuator6.normalizedScopeValues.command,actuatorPlot.actuator6.displayValues.actual,actuatorPlot.actuator6.displayValues.command,actuatorPlot.actuator7.asciiLabel,actuatorPlot.actuator7.normalizedScopeValues.actual,actuatorPlot.actuator7.normalizedScopeValues.command,actuatorPlot.actuator7.displayValues.actual,actuatorPlot.actuator7.displayValues.command,actuatorPlot.actuator8.asciiLabel,actuatorPlot.actuator8.normalizedScopeValues.actual,actuatorPlot.actuator8.normalizedScopeValues.command,actuatorPlot.actuator8.displayValues.actual,actuatorPlot.actuator8.displayValues.command
  Demux : Demux  Outputs=8
  Demux1 : Demux  Outputs=16
  RCD2 Command Empty Bus : $bdroot/To RCD2/RCD2 Command Empty Bus
  Out1 : Outport
  wires:
  Demux1/6 -> Bus Assignment/16
  Demux1/10 -> Bus Assignment/20
  Demux1/4 -> Bus Assignment/14
  Demux1/11 -> Bus Assignment/21
  Demux1/12 -> Bus Assignment/22
  Demux1/3 -> Bus Assignment/13
  In16/1 -> Bus Assignment/38
  In56/1 -> Bus Assignment/78
  Demux/8 -> Bus Assignment/10
  Demux1/8 -> Bus Assignment/18
  Demux1/5 -> Bus Assignment/15
  Bus Assignment/1 -> Out1/1
  In42/1 -> Bus Assignment/64
  In23/1 -> Bus Assignment/45
  In19/1 -> Bus Assignment/41
  Demux1/13 -> Bus Assignment/23
  Demux/3 -> Bus Assignment/5
  Demux/6 -> Bus Assignment/8
  In36/1 -> Bus Assignment/58
  In28/1 -> Bus Assignment/50
  In68/1 -> Bus Assignment/90
  Demux/1 -> Bus Assignment/3
  In30/1 -> Bus Assignment/52
  In38/1 -> Bus Assignment/60
  Demux1/14 -> Bus Assignment/24
  In63/1 -> Bus Assignment/85
  In35/1 -> Bus Assignment/57
  In14/1 -> Bus Assignment/36
  In8/1 -> Bus Assignment/30
  Demux1/15 -> Bus Assignment/25
  Demux/2 -> Bus Assignment/4
  In40/1 -> Bus Assignment/62
  In64/1 -> Bus Assignment/86
  Demux1/16 -> Bus Assignment/26
  In50/1 -> Bus Assignment/72
  Demux1/2 -> Bus Assignment/12
  In47/1 -> Bus Assignment/69
  In13/1 -> Bus Assignment/35
  In34/1 -> Bus Assignment/56
  In43/1 -> Bus Assignment/65
  In15/1 -> Bus Assignment/37
  Demux1/7 -> Bus Assignment/17
  In59/1 -> Bus Assignment/81
  Demux1/1 -> Bus Assignment/11
  Demux/5 -> Bus Assignment/7
  Demux/7 -> Bus Assignment/9
  In31/1 -> Bus Assignment/53
  Demux1/9 -> Bus Assignment/19
  In65/1 -> Bus Assignment/87
  In6/1 -> Bus Assignment/28
  In9/1 -> Bus Assignment/31
  Demux/4 -> Bus Assignment/6
  In53/1 -> Bus Assignment/75
  In61/1 -> Bus Assignment/83
  In57/1 -> Bus Assignment/79
  In18/1 -> Bus Assignment/40
  In7/1 -> Bus Assignment/29
  In20/1 -> Bus Assignment/42
  In69/1 -> Bus Assignment/91
  In45/1 -> Bus Assignment/67
  In52/1 -> Bus Assignment/74
  In26/1 -> Bus Assignment/48
  In58/1 -> Bus Assignment/80
  In25/1 -> Bus Assignment/47
  In39/1 -> Bus Assignment/61
  In46/1 -> Bus Assignment/68
  In29/1 -> Bus Assignment/51
  In12/1 -> Bus Assignment/34
  In21/1 -> Bus Assignment/43
  In33/1 -> Bus Assignment/55
  In44/1 -> Bus Assignment/66
  In24/1 -> Bus Assignment/46
  In62/1 -> Bus Assignment/84
  In41/1 -> Bus Assignment/63
  In55/1 -> Bus Assignment/77
  In67/1 -> Bus Assignment/89
  In49/1 -> Bus Assignment/71
  In22/1 -> Bus Assignment/44
  In11/1 -> Bus Assignment/33
  In17/1 -> Bus Assignment/39
  In66/1 -> Bus Assignment/88
  In51/1 -> Bus Assignment/73
  In54/1 -> Bus Assignment/76
  In60/1 -> Bus Assignment/82
  In37/1 -> Bus Assignment/59
  In4/1 -> Demux1/1
  In27/1 -> Bus Assignment/49
  In3/1 -> Demux/1
  In32/1 -> Bus Assignment/54
  In48/1 -> Bus Assignment/70
  In5/1 -> Bus Assignment/27
  In10/1 -> Bus Assignment/32
  In1/1 -> Bus Assignment/2
  RCD2 Command Empty Bus/1 -> Bus Assignment/1

== system RCD2/To RCD2/RCD2 Command Unpack/Unpack Message/u16 to bitfield ==
  u16 : Inport
  Bitwise AND{6,10..16} (8 alike) : simulink/Logic and Bit Operations/Bitwise Operator  logicop=AND  UseBitMask=on  BitMask=3  BitMaskRealWorld=Stored Integer
      settings: LibrarySourceBlock=|
      | simulink/Quick Insert/Logic and Bit
      | Operations/Bitwise AND
  Data Type Conversion5 : DataTypeConversion  OutDataTypeStr=uint8  SaturateOnIntegerOverflow=off  RndMeth=Floor
  Mux : Mux  Inputs=8
  Shift Arithmetic16 : ArithShift  BitShiftNumber=2  BitShiftDirection=Right
  Shift Arithmetic17 : ArithShift  BitShiftNumber=4  BitShiftDirection=Right
  Shift Arithmetic18 : ArithShift  BitShiftNumber=6  BitShiftDirection=Right
  Shift Arithmetic19 : ArithShift  BitShiftNumber=8  BitShiftDirection=Right
  Shift Arithmetic20 : ArithShift  BitShiftNumber=10  BitShiftDirection=Right
  Shift Arithmetic21 : ArithShift  BitShiftNumber=12  BitShiftDirection=Right
  Shift Arithmetic22 : ArithShift  BitShiftNumber=14  BitShiftDirection=Right
  "bitfield " : Outport
  wires:
  Mux/1 -> Data Type Conversion5/1
  Shift Arithmetic20/1 -> Bitwise AND14/1
  Shift Arithmetic19/1 -> Bitwise AND13/1
  Shift Arithmetic17/1 -> Bitwise AND11/1
  Shift Arithmetic16/1 -> Bitwise AND10/1
  Shift Arithmetic21/1 -> Bitwise AND15/1
  Shift Arithmetic22/1 -> Bitwise AND16/1
  Shift Arithmetic18/1 -> Bitwise AND12/1
  u16/1 -> Shift Arithmetic16/1, Shift Arithmetic17/1, Shift Arithmetic18/1, Shift Arithmetic19/1, Shift Arithmetic20/1, Shift Arithmetic21/1, Shift Arithmetic22/1, Bitwise AND6/1
  Bitwise AND6/1 -> Mux/1
  Bitwise AND10/1 -> Mux/2
  Bitwise AND11/1 -> Mux/3
  Bitwise AND12/1 -> Mux/4
  Bitwise AND13/1 -> Mux/5
  Bitwise AND14/1 -> Mux/6
  Bitwise AND15/1 -> Mux/7
  Bitwise AND16/1 -> Mux/8
  Data Type Conversion5/1 -> "bitfield "/1

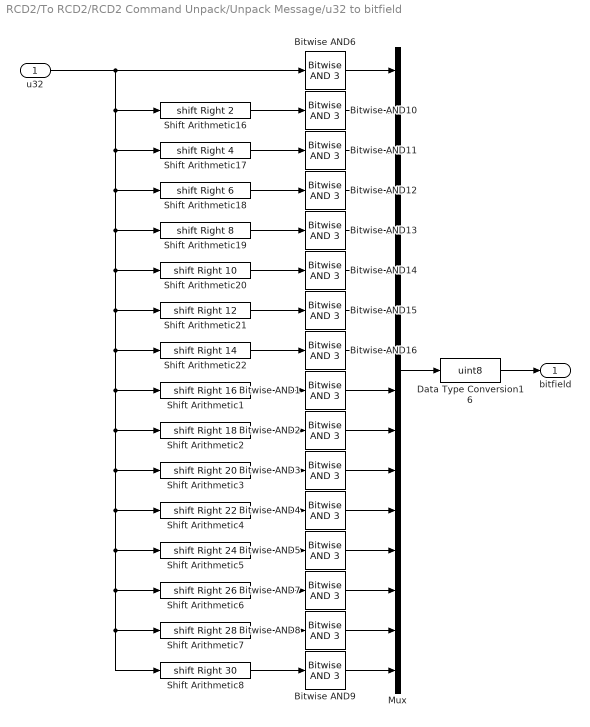
== system RCD2/To RCD2/RCD2 Command Unpack/Unpack Message/u32 to bitfield ==
  u32 : Inport
  Bitwise AND{1..16} (16 alike) : simulink/Logic and Bit Operations/Bitwise Operator  logicop=AND  UseBitMask=on  BitMask=3  BitMaskRealWorld=Stored Integer
      settings: LibrarySourceBlock=|
      | simulink/Quick Insert/Logic and Bit
      | Operations/Bitwise AND
  Data Type Conversion16 : DataTypeConversion  OutDataTypeStr=uint8  SaturateOnIntegerOverflow=off  RndMeth=Floor
  Mux : Mux  Inputs=16
  Shift Arithmetic1 : ArithShift  BitShiftNumber=16  BitShiftDirection=Right
  Shift Arithmetic16 : ArithShift  BitShiftNumber=2  BitShiftDirection=Right
  Shift Arithmetic17 : ArithShift  BitShiftNumber=4  BitShiftDirection=Right
  Shift Arithmetic18 : ArithShift  BitShiftNumber=6  BitShiftDirection=Right
  Shift Arithmetic19 : ArithShift  BitShiftNumber=8  BitShiftDirection=Right
  Shift Arithmetic2 : ArithShift  BitShiftNumber=18  BitShiftDirection=Right
  Shift Arithmetic20 : ArithShift  BitShiftNumber=10  BitShiftDirection=Right
  Shift Arithmetic21 : ArithShift  BitShiftNumber=12  BitShiftDirection=Right
  Shift Arithmetic22 : ArithShift  BitShiftNumber=14  BitShiftDirection=Right
  Shift Arithmetic3 : ArithShift  BitShiftNumber=20  BitShiftDirection=Right
  Shift Arithmetic4 : ArithShift  BitShiftNumber=22  BitShiftDirection=Right
  Shift Arithmetic5 : ArithShift  BitShiftNumber=24  BitShiftDirection=Right
  Shift Arithmetic6 : ArithShift  BitShiftNumber=26  BitShiftDirection=Right
  Shift Arithmetic7 : ArithShift  BitShiftNumber=28  BitShiftDirection=Right
  Shift Arithmetic8 : ArithShift  BitShiftNumber=30  BitShiftDirection=Right
  "bitfield " : Outport
  wires:
  Mux/1 -> Data Type Conversion16/1
  Bitwise AND9/1 -> Mux/16
  Shift Arithmetic8/1 -> Bitwise AND9/1
  Shift Arithmetic7/1 -> Bitwise AND8/1
  Shift Arithmetic6/1 -> Bitwise AND7/1
  Shift Arithmetic5/1 -> Bitwise AND5/1
  Shift Arithmetic4/1 -> Bitwise AND4/1
  Shift Arithmetic3/1 -> Bitwise AND3/1
  Shift Arithmetic2/1 -> Bitwise AND2/1
  Shift Arithmetic1/1 -> Bitwise AND1/1
  Shift Arithmetic18/1 -> Bitwise AND12/1
  Shift Arithmetic22/1 -> Bitwise AND16/1
  Shift Arithmetic21/1 -> Bitwise AND15/1
  Shift Arithmetic16/1 -> Bitwise AND10/1
  Shift Arithmetic17/1 -> Bitwise AND11/1
  Shift Arithmetic19/1 -> Bitwise AND13/1
  Shift Arithmetic20/1 -> Bitwise AND14/1
  u32/1 -> Shift Arithmetic16/1, Shift Arithmetic17/1, Shift Arithmetic18/1, Shift Arithmetic19/1, Shift Arithmetic20/1, Shift Arithmetic21/1, Shift Arithmetic22/1, Shift Arithmetic1/1, Shift Arithmetic2/1, Shift Arithmetic3/1, Shift Arithmetic4/1, Shift Arithmetic5/1, Shift Arithmetic6/1, Shift Arithmetic7/1, Shift Arithmetic8/1, Bitwise AND6/1
  Bitwise AND6/1 -> Mux/1
  Bitwise AND10/1 -> Mux/2
  Bitwise AND11/1 -> Mux/3
  Bitwise AND12/1 -> Mux/4
  Bitwise AND13/1 -> Mux/5
  Bitwise AND14/1 -> Mux/6
  Bitwise AND15/1 -> Mux/7
  Bitwise AND16/1 -> Mux/8
  Bitwise AND1/1 -> Mux/9
  Bitwise AND2/1 -> Mux/10
  Bitwise AND3/1 -> Mux/11
  Bitwise AND4/1 -> Mux/12
  Bitwise AND5/1 -> Mux/13
  Bitwise AND7/1 -> Mux/14
  Bitwise AND8/1 -> Mux/15
  Data Type Conversion16/1 -> "bitfield "/1
